simulink model "Record_accelerometer"  (R2014a)
settings: Solver=FixedStepDiscrete  StartTime=0.0  StopTime=300  FixedStep=1/400  RelTol=1e-3
undefined symbols (not defined in the file or in its folder): DiscIntNeverNeededParam
libraries: simulink x6, aerolibtransform2 x4, vrlib x3, aerolibutil x2, AR_Drone_2_Library x1, dspmtrx3 x1, Navigation_Lib x1
(part 1 of 2)
settings Model: SimulationMode=external  ExtModeTrigDuration=120003  Creator=darenlee  LastModifiedBy=darenlee
settings OptimizationCC: OptimizeModelRefInitCode=on  LifeSpan=1  MaxStackSize=64
settings DebuggingCC: UnderspecifiedInitializationDetection=Classic
settings HardwareCC: ProdLargestAtomicInteger=Long  ProdLargestAtomicFloat=Double  ProdEndianess=LittleEndian  ProdHWDeviceType=ARM Compatible->ARM Cortex
settings RTWCC: SystemTargetFile=ert.tlc  TLCOptions=-aInlineSetEventsForThisBaseRateFcn=TLC_FALSE -aSuppressMultiTaskScheduler=TLC_FALSE  TemplateMakefile=ert_default_tmf  Description=Embedded Coder  ProcessScript=ert_make_rtw_hook  Toolchain=Code Sourcery
settings CodeAppCC: IgnoreCustomStorageClasses=off
settings ERTTargetCC: ParMdlRefBuildCompliant=on  CompOptLevelCompliant=on  ConcurrentExecutionCompliant=on  ERTFirstTimeCompliant=on  ModelStepFunctionPrototypeControlCompliant=on  CPPClassGenCompliant=on  ExtMode=on  ExtModeMexArgs='192.168.1.1' 1 17725  InlinedParameterPlacement=Hierarchical

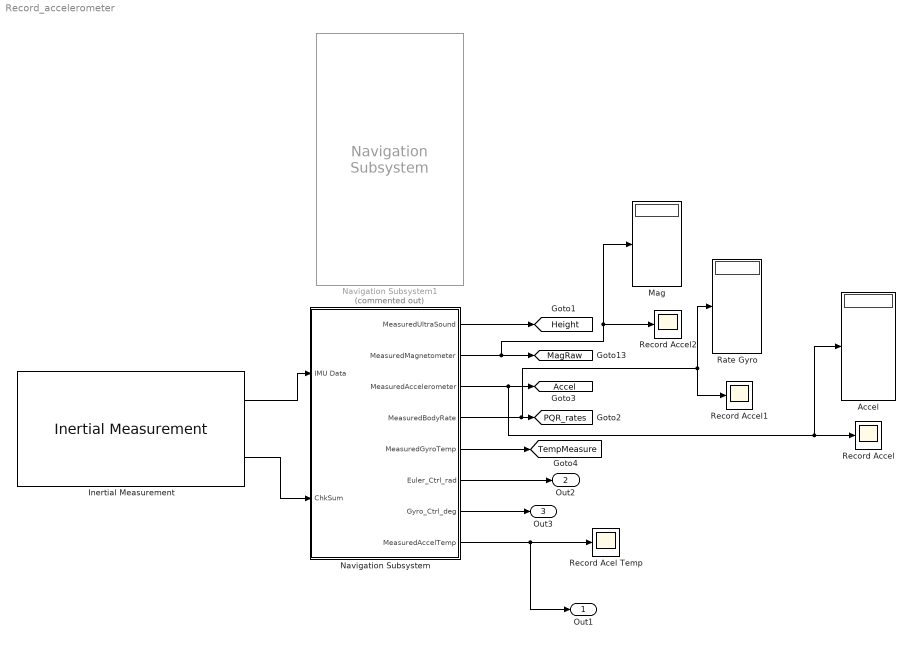
== system Record_accelerometer ==
  Accel : Display
  Inertial Measurement : AR_Drone_2_Library/Inertial Measurement  Ts=1/400
  Mag : Display
  Navigation Subsystem : Subsystem
  Navigation Subsystem1 : Navigation_Lib/Navigation Subsystem  Commented=on  TempProcessVariant=1  PI_YAW_CORRECT=[-0.9 -0.0001]  D_YAW_CORRECT=0  P_GAIN_ROLLPITCH=-2  I_GAIN_ROLLPITCH=-0.01  ACCEL_OFFSET_X=0  ACCEL_OFFSET_Y=0  ACCEL_OFFSET_Z=0
  Rate Gyro : Display
  Record Accel : Scope
      settings: YMin=1550  YMax=2050  SaveName=Accel_Record
  Record Accel1 : Scope
      settings: YMin=1550  YMax=2050  SaveName=Accel_Record1
  Record Accel2 : Scope
      settings: YMin=1550  YMax=2050  SaveName=Accel_Record2
  Record Acel Temp : Scope
      settings: SaveName=Accel_temp
  Out1 : Outport
  Out2 : Outport  Port=2
  Out3 : Outport  Port=3
  tag scope: Accel=global, Height=global, MagRaw=global, PQR_rates=global, TempMeasure=global
  wires:
  Inertial Measurement/1 -> Navigation Subsystem/1(IMU Data)
  Inertial Measurement/2 -> Navigation Subsystem/2(ChkSum)
  Navigation Subsystem/1(MeasuredUltraSound) -> [Height]
  Navigation Subsystem/2(MeasuredMagnetometer) -> Mag/1, Record Accel2/1, [MagRaw]
  Navigation Subsystem/3(MeasuredAccelerometer) -> Accel/1, Record Accel/1, [Accel]
  Navigation Subsystem/4(MeasuredBodyRate) -> Record Accel1/1, Rate Gyro/1, [PQR_rates]
  Navigation Subsystem/5(MeasuredGyroTemp) -> [TempMeasure]
  Navigation Subsystem/8(MeasuredAccelTemp) -> Out1/1, Record Acel Temp/1
  Navigation Subsystem/6(Euler_Ctrl_rad) -> Out2/1
  Navigation Subsystem/7(Gyro_Ctrl_deg) -> Out3/1

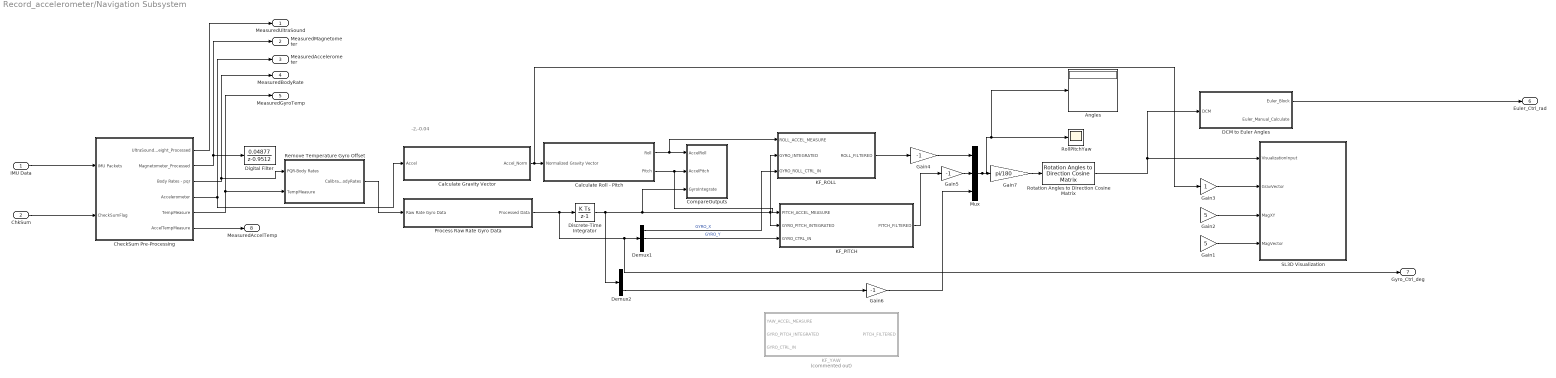
== system Record_accelerometer/Navigation Subsystem ==
  note: -2,-0.04
  IMU Data : Inport
  ChkSum : Inport  Port=2
  Angles : Display
  Calculate Gravity Vector : Subsystem
  Calculate Roll - Pitch : Subsystem
  CheckSum Pre-Processing : Subsystem
  CompareOutputs : Subsystem
  DCM to Euler Angles : Subsystem
  Demux1 : Demux  Outputs=3
  Demux2 : Demux  Outputs=3
  Digital Filter : DiscreteTransferFcn  Numerator=[0.04877]  Denominator=[1 -0.9512]  SampleTime=1/400
  Discrete-Time Integrator : DiscreteIntegrator  SampleTime=1/400  ICPrevOutput=DiscIntNeverNeededParam  ICPrevScaledInput=DiscIntNeverNeededParam
  Gain1 : Gain  Gain=5  OutDataTypeStr=double
  Gain2 : Gain  Gain=5  OutDataTypeStr=double
  Gain3 : Gain  OutDataTypeStr=double
  Gain4 : Gain  Gain=-1
  Gain5 : Gain  Gain=-1
  Gain6 : Gain  Gain=-1
  Gain7 : Gain  Gain=pi/180
  KF_PITCH : Subsystem
  KF_ROLL : Subsystem
  KF_YAW : Subsystem  Commented=on
  Mux : Mux  Inputs=3
  Process Raw Rate Gyro Data : Subsystem
  Remove Temperature Gyro Offset : Subsystem  Variant=on  OverrideUsingVariant=TempConditionA
  RollPitchYaw : Scope
      settings: YMin=0  YMax=70  SaveName=ScopeData15
  Rotation Angles to Direction Cosine Matrix : aerolibtransform2/Rotation Angles to Direction Cosine Matrix  rotationOrder=XYZ
  SL3D Visualization : Subsystem
  MeasuredUltraSound : Outport
  MeasuredMagnetometer : Outport  Port=2
  MeasuredAccelerometer : Outport  Port=3
  MeasuredBodyRate : Outport  Port=4
  MeasuredGyroTemp : Outport  Port=5
  Euler_Ctrl_rad : Outport  Port=6
  Gyro_Ctrl_deg : Outport  Port=7
  MeasuredAccelTemp : Outport  Port=8
  wires:
  IMU Data/1 -> CheckSum Pre-Processing/1(IMU Packets)
  ChkSum/1 -> CheckSum Pre-Processing/2(CheckSumFlag)
  CheckSum Pre-Processing/1(UltraSoundHeight_Processed) -> MeasuredUltraSound/1
  CheckSum Pre-Processing/4(Accelerometer) -> Calculate Gravity Vector/1(Accel), MeasuredAccelerometer/1
  CheckSum Pre-Processing/3(Body Rates - pqr) -> MeasuredBodyRate/1, Remove Temperature Gyro Offset/1(PQR-Body Rates)
  CheckSum Pre-Processing/2(Magnetometer_Processed) -> MeasuredMagnetometer/1, Digital Filter/1
  CheckSum Pre-Processing/5(TempMeasure) -> MeasuredGyroTemp/1, Remove Temperature Gyro Offset/2(TempMeasure)
  Remove Temperature Gyro Offset/1(Calibrated-BodyRates) -> Process Raw Rate Gyro Data/1(Raw Rate Gyro Data)
  Rotation Angles to Direction Cosine Matrix/1 -> SL3D Visualization/1(VisualizationInput), DCM to Euler Angles/1(DCM)
  Gain1/1 -> SL3D Visualization/4(MagVector)
  Gain2/1 -> SL3D Visualization/3(MagXY)
  Calculate Gravity Vector/1(Accel_Norm) -> Gain3/1, Calculate Roll - Pitch/1(Normalized Gravity Vector)
  Gain3/1 -> SL3D Visualization/2(GravVector)
  ? -> Gain1/1
  ? -> Gain2/1
  Mux/1 -> RollPitchYaw/1, Angles/1, Gain7/1
  Process Raw Rate Gyro Data/1(Processed Data) -> Gyro_Ctrl_deg/1, Demux1/1, Discrete-Time Integrator/1
  Calculate Roll - Pitch/1(Roll) -> KF_ROLL/1(ROLL_ACCEL_MEASURE), CompareOutputs/1(AccelRoll)
  Calculate Roll - Pitch/2(Pitch) -> KF_PITCH/1(PITCH_ACCEL_MEASURE), CompareOutputs/2(AccelPitch)
  Discrete-Time Integrator/1 -> CompareOutputs/3(GyroIntegrate), KF_PITCH/2(GYRO_PITCH_INTEGRATED), KF_ROLL/2(GYRO_INTEGRATED), Demux2/1
  Demux1/1 -> KF_ROLL/3(GYRO_ROLL_CTRL_IN)  "GYRO_X"
  Demux1/2 -> KF_PITCH/3(GYRO_CTRL_IN)  "GYRO_Y"
  KF_ROLL/1(ROLL_FILTERED) -> Gain4/1
  KF_PITCH/1(PITCH_FILTERED) -> Gain5/1
  Gain6/1 -> Mux/3
  Gain7/1 -> Rotation Angles to Direction Cosine Matrix/1
  Gain4/1 -> Mux/1
  Gain5/1 -> Mux/2
  Demux2/3 -> Gain6/1
  DCM to Euler Angles/1(Euler_Block) -> Euler_Ctrl_rad/1
  CheckSum Pre-Processing/6(AccelTempMeasure) -> MeasuredAccelTemp/1

== system Record_accelerometer/Navigation Subsystem/Calculate Gravity Vector ==
  Accel : Inport
  Accelerometer Neutral Gain and Offset : Subsystem
  Low Pass Filter : Subsystem
  New Dead Zone Method : Subsystem
  Normalize Vector : vrlib/Utilities/Normalize Vector  Commented=through  maxzero=0
  Old Offset Method : Subsystem
  Scope : Scope
      settings: YMin=-1  YMax=0.05  SaveName=ScopeData11
  Scope1 : Scope  NumInputPorts=2
      settings: TimeRange=6.848856838354834  YMin=-1.05~-1  YMax=0.05~0.05  SaveName=AccelProcessed_Record
  Accel_Norm : Outport
  wires:
  Normalize Vector/1 -> Accel_Norm/1
  Accel/1 -> Accelerometer Neutral Gain and Offset/1(Raw Accel Data)
  Accelerometer Neutral Gain and Offset/1(Processed Accel Data) -> Old Offset Method/1(In1), Scope1/2
  Old Offset Method/1(Out1) -> Scope1/1, Low Pass Filter/1(Offset Accel)
  Low Pass Filter/1(Filtered Accel) -> Normalize Vector/1, Scope/1

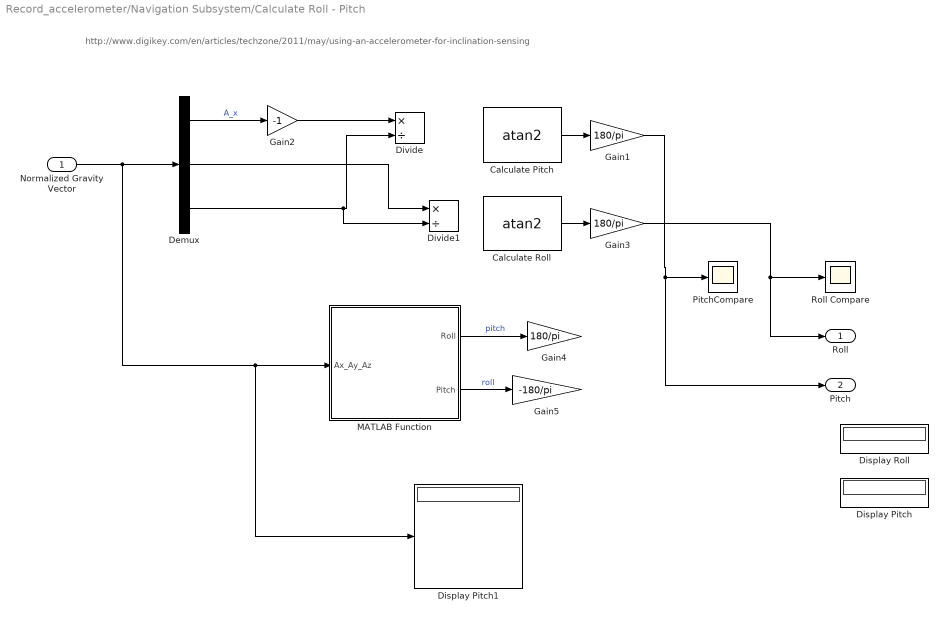
== system Record_accelerometer/Navigation Subsystem/Calculate Roll - Pitch ==
  note: http://www.digikey.com/en/articles/techzone/2011/may/using-an-accelerometer-for-inclination-sensing
  Normalized Gravity Vector : Inport
  Calculate Pitch : Trigonometry  Operator=atan2
  Calculate Roll : Trigonometry  Operator=atan2
  Demux : Demux  Outputs=3
  Display Pitch : Display
  Display Pitch1 : Display
  Display Roll : Display
  Divide : Product  Inputs=*/
  Divide1 : Product  Inputs=*/
  Gain1 : Gain  Gain=180/pi
  Gain2 : Gain  Gain=-1
  Gain3 : Gain  Gain=180/pi
  Gain4 : Gain  Gain=180/pi
  Gain5 : Gain  Gain=-180/pi
  MATLAB Function : MATLAB Function  TreatAsAtomicUnit=on
  PitchCompare : Scope
      settings: YMin=0  YMax=3.25  SaveName=ScopeData9
  Roll Compare : Scope
      settings: TimeRange=30  YMin=-2.175  YMax=-1.7  SaveName=ScopeData5
  Roll : Outport
  Pitch : Outport  Port=2
  wires:
  Calculate Pitch/1 -> Gain1/1
  Calculate Roll/1 -> Gain3/1
  Demux/1 -> Gain2/1  "A_x"
  Normalized Gravity Vector/1 -> Display Pitch1/1, MATLAB Function/1(Ax_Ay_Az), Demux/1
  MATLAB Function/1(Roll) -> Gain4/1  "pitch"
  MATLAB Function/2(Pitch) -> Gain5/1  "roll"
  Gain1/1 -> PitchCompare/1, Pitch/1
  Gain3/1 -> Roll Compare/1, Roll/1
  Demux/2 -> Divide1/1
  Gain2/1 -> Divide/1
  Demux/3 -> Divide1/2, Divide/2

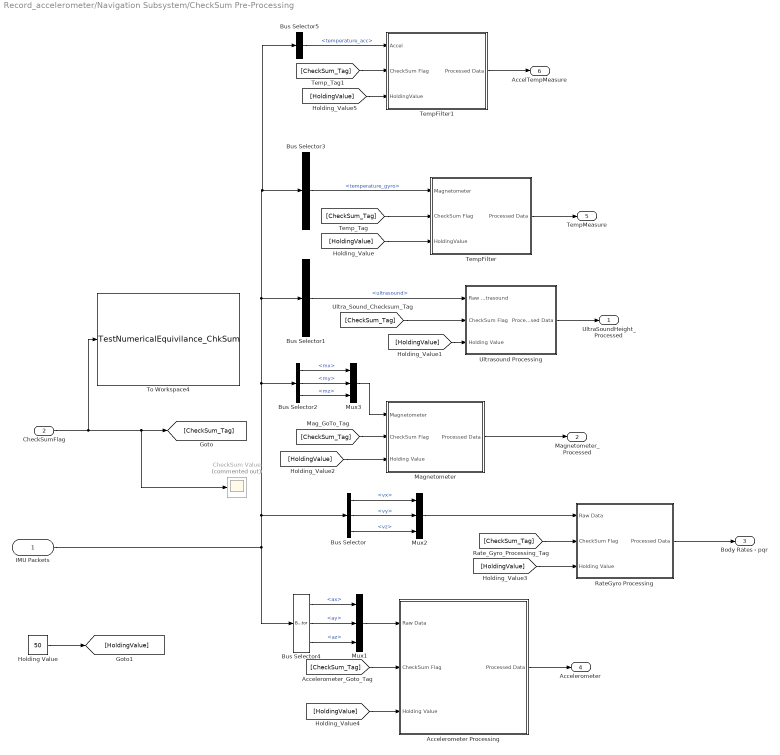
== system Record_accelerometer/Navigation Subsystem/CheckSum Pre-Processing ==
  IMU Packets : Inport
  CheckSumFlag : Inport  Port=2
  Accelerometer Processing : Subsystem
  Bus Selector : BusSelector  OutputSignals=vx,vy,vz
  Bus Selector1 : BusSelector  OutputSignals=ultrasound
  Bus Selector2 : BusSelector  OutputSignals=mx,my,mz
  Bus Selector3 : BusSelector  OutputSignals=temperature_gyro
  Bus Selector4 : BusSelector  OutputSignals=ax,ay,az
  Bus Selector5 : BusSelector  OutputSignals=temperature_acc
  CheckSum Value : Scope  Commented=on
      settings: YMin=0  YMax=2500  SaveName=CheckSum
  Holding Value : Constant  Value=50
  Magnetometer : Subsystem
  Mux1 : Mux  Inputs=3
  Mux2 : Mux  Inputs=3
  Mux3 : Mux  Inputs=3
  RateGyro Processing : Subsystem
  TempFilter : Subsystem
  TempFilter1 : Subsystem
  To Workspace4 : ToWorkspace  VariableName=TestNumericalEquivilance_ChkSum  SaveFormat=Structure With Time  SampleTime=-1
  Ultrasound Processing : Subsystem
  UltraSoundHeight_Processed : Outport
  Magnetometer_Processed : Outport  Port=2
  Body Rates - pqr : Outport  Port=3
  Accelerometer : Outport  Port=4
  TempMeasure : Outport  Port=5
  AccelTempMeasure : Outport  Port=6
  wires:
  Bus Selector1/1 -> Ultrasound Processing/1(Raw Ultrasound)  "<ultrasound>"
  CheckSumFlag/1 -> To Workspace4/1, [CheckSum_Tag], CheckSum Value/1
  IMU Packets/1 -> Bus Selector/1, Bus Selector5/1, Bus Selector3/1, Bus Selector1/1, Bus Selector2/1, Bus Selector4/1
  Bus Selector4/1 -> Mux1/1  "<ax>"
  Bus Selector4/2 -> Mux1/2  "<ay>"
  Bus Selector4/3 -> Mux1/3  "<az>"
  Mux1/1 -> Accelerometer Processing/1(Raw Data)
  [CheckSum_Tag] -> Ultrasound Processing/2(CheckSum Flag)
  Accelerometer Processing/1(Processed Data) -> Accelerometer/1
  Mux2/1 -> RateGyro Processing/1(Raw Data)
  [CheckSum_Tag] -> RateGyro Processing/2(CheckSum Flag)
  RateGyro Processing/1(Processed Data) -> Body Rates - pqr/1
  Bus Selector2/1 -> Mux3/1  "<mx>"
  Bus Selector2/2 -> Mux3/2  "<my>"
  Bus Selector2/3 -> Mux3/3  "<mz>"
  [CheckSum_Tag] -> Magnetometer/2(CheckSum Flag)
  Magnetometer/1(Processed Data) -> Magnetometer_Processed/1
  [CheckSum_Tag] -> Accelerometer Processing/2(CheckSum Flag)
  Ultrasound Processing/1(Processed Data) -> UltraSoundHeight_Processed/1
  Bus Selector/1 -> Mux2/1  "<vx>"
  Bus Selector/2 -> Mux2/2  "<vy>"
  Bus Selector/3 -> Mux2/3  "<vz>"
  Bus Selector3/1 -> TempFilter/1(Magnetometer)  "<temperature_gyro>"
  TempFilter/1(Processed Data) -> TempMeasure/1
  [CheckSum_Tag] -> TempFilter/2(CheckSum Flag)
  [HoldingValue] -> TempFilter/3(HoldingValue)
  [HoldingValue] -> Ultrasound Processing/3(Holding Value)
  [HoldingValue] -> Magnetometer/3(Holding Value)
  [HoldingValue] -> RateGyro Processing/3(Holding Value)
  [HoldingValue] -> Accelerometer Processing/3(Holding Value)
  Holding Value/1 -> [HoldingValue]
  Mux3/1 -> Magnetometer/1(Magnetometer)
  TempFilter1/1(Processed Data) -> AccelTempMeasure/1
  [CheckSum_Tag] -> TempFilter1/2(CheckSum Flag)
  [HoldingValue] -> TempFilter1/3(HoldingValue)
  Bus Selector5/1 -> TempFilter1/1(Accel)  "<temperature_acc>"

== system Record_accelerometer/Navigation Subsystem/CompareOutputs ==
  AccelRoll : Inport
  AccelPitch : Inport  Port=2
  GyroIntegrate : Inport  Port=3
  Demux : Demux  Outputs=3
  Mux : Mux  Inputs=2
  Mux1 : Mux  Inputs=2
  Scope : Scope
      settings: YMin=-3  YMax=14  SaveName=ScopeData7
  Scope1 : Scope
      settings: SaveName=ScopeData8
  wires:
  AccelPitch/1 -> Mux1/1
  Demux/2 -> Mux1/2
  AccelRoll/1 -> Mux/1
  Demux/1 -> Mux/2
  GyroIntegrate/1 -> Demux/1
  Mux/1 -> Scope/1
  Mux1/1 -> Scope1/1

== system Record_accelerometer/Navigation Subsystem/DCM to Euler Angles ==
  note: Euler Rotation Order:
      | With the camera facing towards you
      | ______________
      |       Camera          |
      | 1                    2    |
      |                             |
      | 3                    4    |
      | ______________|
      |
      | Rotation
      |
      | Roll+ , increase 2+4
      | Roll - , increase 1 3
      |
      | Pitch+ , increaes 1+2
      | Pitch- , increase 3+4
  DCM : Inport
  Constant2 : Constant  Value=[1 0 0]
  Direction Cosine Matrix to Rotation Angles : aerolibtransform2/Direction Cosine Matrix to Rotation Angles  rotationOrder=XYZ  lim=Default
      settings: AttributesFormatString=Rotation Order: %<rotationOrder>
  EulerAnglesCalculation : Subsystem  TreatAsAtomicUnit=on
  Product : Product  Multiplication=Matrix(*)
  VectorTrace : Scope
      settings: SaveName=RotationVectorTrace
  Euler_Block : Outport
  Euler_Manual_Calculate : Outport  Port=2
  wires:
  DCM/1 -> Direction Cosine Matrix to Rotation Angles/1, Product/1, EulerAnglesCalculation/1(DCM)
  EulerAnglesCalculation/1(Euler Angles) -> Euler_Manual_Calculate/1
  Direction Cosine Matrix to Rotation Angles/1 -> Euler_Block/1
  Constant2/1 -> Product/2
  Product/1 -> VectorTrace/1

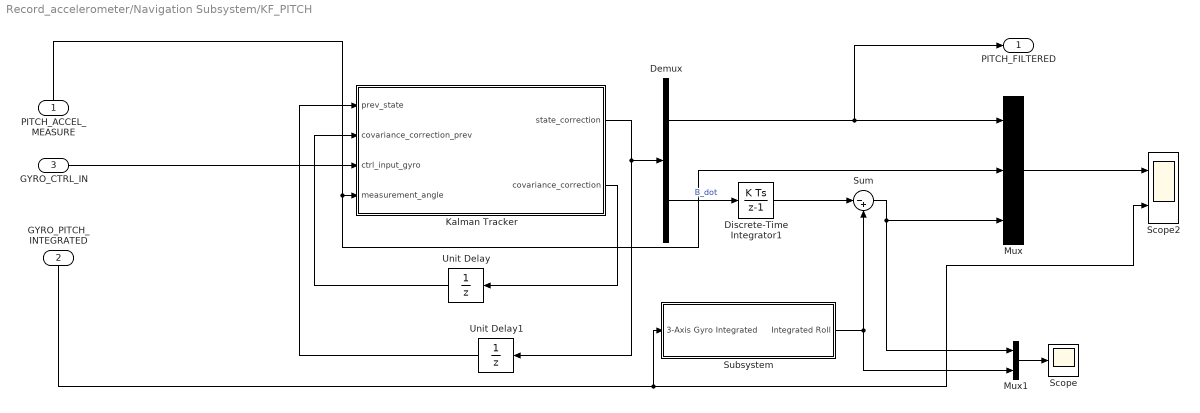
== system Record_accelerometer/Navigation Subsystem/KF_PITCH ==
  PITCH_ACCEL_MEASURE : Inport
  GYRO_PITCH_INTEGRATED : Inport  Port=2
  GYRO_CTRL_IN : Inport  Port=3
  Demux : Demux  Outputs=2
  Discrete-Time Integrator1 : DiscreteIntegrator  SampleTime=1/400  ICPrevOutput=DiscIntNeverNeededParam  ICPrevScaledInput=DiscIntNeverNeededParam
  Kalman Tracker : MATLAB Function  TreatAsAtomicUnit=on
  Mux : Mux  Inputs=3
  Mux1 : Mux  Inputs=2
  Scope : Scope
      settings: YMin=0.05  YMax=1.05  SaveName=ScopeData14
  Scope2 : Scope  NumInputPorts=2
      settings: YMin=0~-90  YMax=30~5  SaveName=ScopeData10
  Subsystem : Subsystem
  Sum : Sum  Inputs=|-+
  Unit Delay : UnitDelay  InitialCondition=eye(2)  SampleTime=-1
  Unit Delay1 : UnitDelay  InitialCondition=[0 0]'  SampleTime=-1
  PITCH_FILTERED : Outport
  wires:
  Mux1/1 -> Scope/1
  Discrete-Time Integrator1/1 -> Sum/1
  Demux/2 -> Discrete-Time Integrator1/1  "B_dot"
  Sum/1 -> Mux1/1, Mux/3
  Subsystem/1(Integrated Roll) -> Mux1/2, Sum/2
  Kalman Tracker/2(covariance_correction) -> Unit Delay/1
  Demux/1 -> PITCH_FILTERED/1, Mux/1
  Kalman Tracker/1(state_correction) -> Unit Delay1/1, Demux/1
  Mux/1 -> Scope2/1
  Unit Delay1/1 -> Kalman Tracker/1(prev_state)
  GYRO_CTRL_IN/1 -> Kalman Tracker/3(ctrl_input_gyro)
  Unit Delay/1 -> Kalman Tracker/2(covariance_correction_prev)
  GYRO_PITCH_INTEGRATED/1 -> Scope2/2, Subsystem/1(3-Axis Gyro Integrated)
  PITCH_ACCEL_MEASURE/1 -> Mux/2, Kalman Tracker/4(measurement_angle)

== system Record_accelerometer/Navigation Subsystem/KF_ROLL ==
  ROLL_ACCEL_MEASURE : Inport
  GYRO_INTEGRATED : Inport  Port=2
  GYRO_ROLL_CTRL_IN : Inport  Port=3
  Demux : Demux  Outputs=2
  Discrete-Time Integrator1 : DiscreteIntegrator  SampleTime=1/400  ICPrevOutput=DiscIntNeverNeededParam  ICPrevScaledInput=DiscIntNeverNeededParam
  Kalman Tracker : MATLAB Function  TreatAsAtomicUnit=on
  Mux : Mux  Inputs=3
  Mux1 : Mux  Inputs=2
  Scope : Scope
      settings: YMin=0.05  YMax=1.05  SaveName=ScopeData14
  Scope2 : Scope  NumInputPorts=2
      settings: YMin=-20.1~-15  YMax=-18~1  SaveName=ScopeData10
  Subsystem : Subsystem
  Sum : Sum  Inputs=|-+
  Unit Delay : UnitDelay  InitialCondition=eye(2)  SampleTime=-1
  Unit Delay1 : UnitDelay  InitialCondition=[0 0]'  SampleTime=-1
  ROLL_FILTERED : Outport
  wires:
  Mux1/1 -> Scope/1
  Discrete-Time Integrator1/1 -> Sum/1
  Demux/2 -> Discrete-Time Integrator1/1  "B_dot"
  Sum/1 -> Mux1/1, Mux/3
  Subsystem/1(Integrated Roll) -> Mux1/2, Sum/2
  Kalman Tracker/2(covariance_correction) -> Unit Delay/1
  Kalman Tracker/1(state_correction) -> Unit Delay1/1, Demux/1
  Mux/1 -> Scope2/1
  Unit Delay1/1 -> Kalman Tracker/1(prev_state)
  GYRO_ROLL_CTRL_IN/1 -> Kalman Tracker/3(ctrl_input_gyro)
  Unit Delay/1 -> Kalman Tracker/2(covariance_correction_prev)
  GYRO_INTEGRATED/1 -> Scope2/2, Subsystem/1(3-Axis Gyro Integrated)
  ROLL_ACCEL_MEASURE/1 -> Mux/2, Kalman Tracker/4(measurement_angle)
  Demux/1 -> ROLL_FILTERED/1, Mux/1

== system Record_accelerometer/Navigation Subsystem/KF_YAW ==
  YAW_ACCEL_MEASURE : Inport
  GYRO_PITCH_INTEGRATED : Inport  Port=2
  GYRO_CTRL_IN : Inport  Port=3
  Demux : Demux  Outputs=2
  Discrete-Time Integrator1 : DiscreteIntegrator  SampleTime=1/400  ICPrevOutput=DiscIntNeverNeededParam  ICPrevScaledInput=DiscIntNeverNeededParam
  Kalman Tracker : MATLAB Function  TreatAsAtomicUnit=on
  Mux : Mux  Inputs=3
  Mux1 : Mux  Inputs=2
  Scope : Scope
      settings: YMin=0.05  YMax=1.05  SaveName=ScopeData14
  Scope2 : Scope  NumInputPorts=2
      settings: YMin=0~-90  YMax=30~5  SaveName=ScopeData10
  Subsystem : Subsystem
  Sum : Sum  Inputs=|-+
  Unit Delay : UnitDelay  InitialCondition=eye(2)  SampleTime=-1
  Unit Delay1 : UnitDelay  InitialCondition=[0 0]'  SampleTime=-1
  PITCH_FILTERED : Outport
  wires:
  Mux1/1 -> Scope/1
  Discrete-Time Integrator1/1 -> Sum/1
  Demux/2 -> Discrete-Time Integrator1/1  "B_dot"
  Sum/1 -> PITCH_FILTERED/1, Mux1/1, Mux/3
  Subsystem/1(Integrated Roll) -> Mux1/2, Sum/2
  Kalman Tracker/2(covariance_correction) -> Unit Delay/1
  Demux/1 -> Mux/1
  Kalman Tracker/1(state_correction) -> Unit Delay1/1, Demux/1
  Mux/1 -> Scope2/1
  Unit Delay1/1 -> Kalman Tracker/1(prev_state)
  GYRO_CTRL_IN/1 -> Kalman Tracker/3(ctrl_input_gyro)
  Unit Delay/1 -> Kalman Tracker/2(covariance_correction_prev)
  GYRO_PITCH_INTEGRATED/1 -> Scope2/2, Subsystem/1(3-Axis Gyro Integrated)
  YAW_ACCEL_MEASURE/1 -> Mux/2, Kalman Tracker/4(measurement_angle)

== system Record_accelerometer/Navigation Subsystem/Process Raw Rate Gyro Data ==
  note: const float Sensitivity[ 3 ] = { 0.0609 , 0.0609 , 0.0609 } ;
      | const float Neutral[ 3 ] = { 0.0 , 0.0 , 0.0 } ;
      | const int16_t Offset[ 3 ] = { - 73 , 14 , - 13 } ;
      | const int16_t Noises[ 3 ] = { 35 , 35 , 15 } ;
      |
      | int16_t vRaws[ 3 ] = {
      | Navdata :: IMU :: Gyroscope :: getRawX (),
      | Navdata :: IMU :: Gyroscope :: getRawY (),
      | Navdata :: IMU :: Gyroscope :: getRawZ ()
      | } ;
      |
      | gyroscope[i] = vRaws[i] * Gyroscope :: Sensitivity[i] * M_PI / 180.0 ;
  Raw Rate Gyro Data : Inport
  Constant1 : Constant  Value=0
  Gain : Gain  Gain=[0.0609, 0.0609, 0.0609]
  Sum : Sum  Inputs=|++
  Processed Data : Outport
  wires:
  Sum/1 -> Gain/1
  Gain/1 -> Processed Data/1
  Raw Rate Gyro Data/1 -> Sum/1
  Constant1/1 -> Sum/2

== system Record_accelerometer/Navigation Subsystem/Remove Temperature Gyro Offset ==
  note: 1) Only subsystems can be added as variant choices at this level
      | 2) Blocks cannot be connected at this level as connectivity is
      | automatically determined at simulation, based on the active variant
  PQR-Body Rates : Inport
  TempMeasure : Inport  Port=2
  TemperatureOffset (home_330453) : Subsystem  VariantControl=TempConditionA
  TemperatureOffset (work_255725) : Subsystem  VariantControl=TempConditionB
  Calibrated-BodyRates : Outport

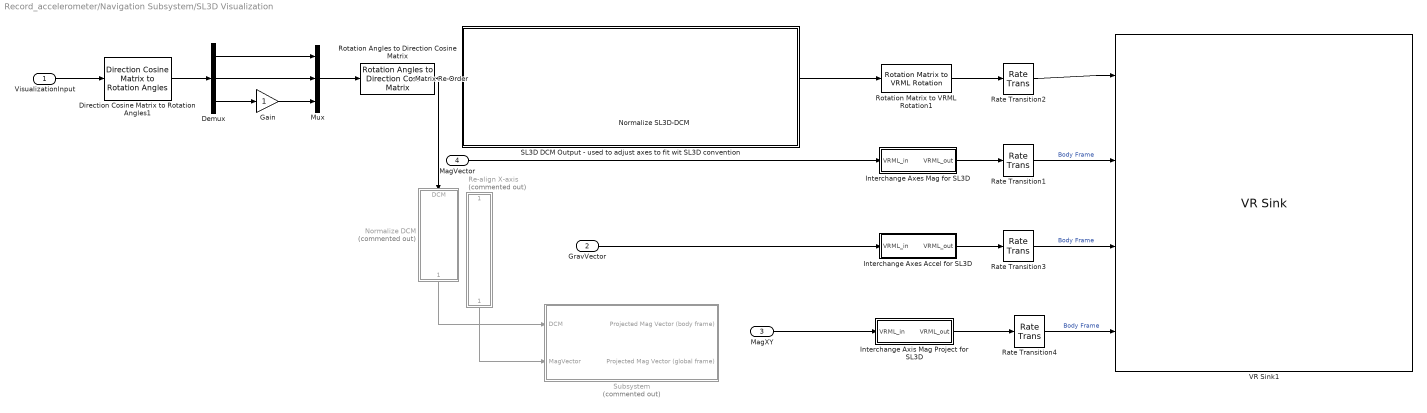
== system Record_accelerometer/Navigation Subsystem/SL3D Visualization ==
  VisualizationInput : Inport
  GravVector : Inport  Port=2
  MagXY : Inport  Port=3
  MagVector : Inport  Port=4
  Demux : Demux  Outputs=3
  Direction Cosine Matrix to Rotation Angles1 : aerolibtransform2/Direction Cosine Matrix to Rotation Angles  rotationOrder=XYZ  lim=ZeroR3
      settings: AttributesFormatString=Rotation Order: %<rotationOrder>
  Gain : Gain  OutDataTypeStr=Inherit: Same as input
  "Interchange Axes Accel for SL3D " : Subsystem
  "Interchange Axes Mag for SL3D " : Subsystem
  Interchange Axis Mag Project for SL3D : Subsystem
  Matrix Re-Order : MATLAB Function  TreatAsAtomicUnit=on
  Mux : Mux  Inputs=3
  Normalize DCM : Subsystem  Commented=on  TreatAsAtomicUnit=on
  Normalize SL3D-DCM : Subsystem  TreatAsAtomicUnit=on
  Rate Transition{1..4} (4 alike) : RateTransition
  Re-align X-axis : Subsystem  Commented=on
  Rotation Angles to Direction Cosine Matrix : aerolibtransform2/Rotation Angles to Direction Cosine Matrix  rotationOrder=XYZ
  Rotation Matrix to VRML Rotation1 : vrlib/Utilities/Rotation Matrix to VRML Rotation  maxzero=1e-12
  SL3D DCM Output - used to adjust axes to fit wit SL3D convention : Subsystem
  Subsystem : Subsystem  Commented=on
  VR Sink1 : vrlib/VR Sink  InstantiateOnLoad=on  SampleTime=0.02  ViewEnable=on  RemoteChange=off  RemoteView=off  FieldsWritten=Plane.rotation.4.1.1.double#mag_point.translation.3.1.1.double#grav_point.translation.3.1.1.double#mag_projection_point.translation.3.1.1.double  WorldFileName=vrml8_grav_2.WRL  AutoView=off  VideoDimensions=[]  AllowVariableSize=off
  wires:
  Rotation Matrix to VRML Rotation1/1 -> Rate Transition2/1
  "Interchange Axes Accel for SL3D "/1(VRML_out) -> Rate Transition3/1
  VisualizationInput/1 -> Direction Cosine Matrix to Rotation Angles1/1
  GravVector/1 -> "Interchange Axes Accel for SL3D "/1(VRML_in)
  Matrix Re-Order/1(M_out) -> Normalize SL3D-DCM/1(DCM)
  Normalize SL3D-DCM/1(DCM_normalized) -> Rotation Matrix to VRML Rotation1/1
  Direction Cosine Matrix to Rotation Angles1/1 -> Demux/1
  Demux/1 -> Mux/1
  Demux/2 -> Mux/2
  Demux/3 -> Gain/1
  Gain/1 -> Mux/3
  Mux/1 -> Rotation Angles to Direction Cosine Matrix/1
  "Interchange Axes Mag for SL3D "/1(VRML_out) -> Rate Transition1/1
  MagVector/1 -> "Interchange Axes Mag for SL3D "/1(VRML_in)
  Rotation Angles to Direction Cosine Matrix/1 -> Matrix Re-Order/1(M_in), Normalize DCM/1(DCM)
  Interchange Axis Mag Project for SL3D/1(VRML_out) -> Rate Transition4/1
  Rate Transition4/1 -> VR Sink1/4  "Body Frame"
  Rate Transition3/1 -> VR Sink1/3  "Body Frame"
  Rate Transition1/1 -> VR Sink1/2  "Body Frame"
  Rate Transition2/1 -> VR Sink1/1
  Normalize DCM/1(DCM_normalized) -> Subsystem/1(DCM)
  Re-align X-axis/1(MagVectorOut) -> Subsystem/2(MagVector)
  MagXY/1 -> Interchange Axis Mag Project for SL3D/1(VRML_in)

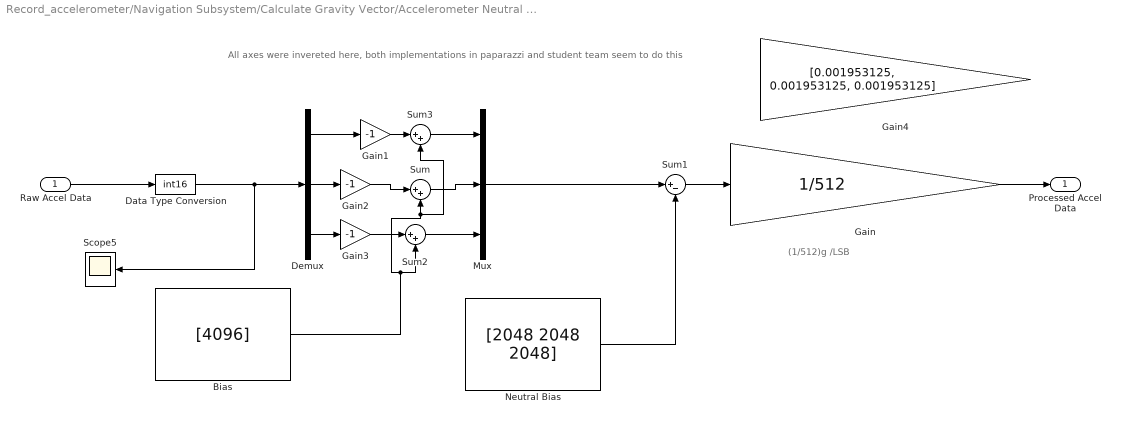
== system Record_accelerometer/Navigation Subsystem/Calculate Gravity Vector/Accelerometer Neutral Gain and Offset ==
  note: All axes were invereted here, both implementations in paparazzi and student team seem to do this
  note: (1/512)g /LSB
  Raw Accel Data : Inport
  Bias : Constant  Value=[4096]
  Data Type Conversion : DataTypeConversion  OutDataTypeStr=int16
  Demux : Demux  Outputs=3
  Gain : Gain  Gain=1/512
  Gain1 : Gain  Gain=-1  OutDataTypeStr=double
  Gain2 : Gain  Gain=-1  OutDataTypeStr=double
  Gain3 : Gain  Gain=-1  OutDataTypeStr=double
  Gain4 : Gain  Gain=[0.001953125, 0.001953125, 0.001953125]
  Mux : Mux  Inputs=3
  Neutral Bias : Constant  Value=[2048 2048 2048]
  Scope5 : Scope
      settings: TimeRange=40  YMin=1530.554926387316  YMax=2010.554926387316  SaveName=ScopeData6
  Sum : Sum  Inputs=|++
  Sum1 : Sum  Inputs=|+-
  Sum2 : Sum  Inputs=|++
  Sum3 : Sum  Inputs=|++
  Processed Accel Data : Outport
  wires:
  Sum1/1 -> Gain/1
  Gain/1 -> Processed Accel Data/1
  Mux/1 -> Sum1/1
  Neutral Bias/1 -> Sum1/2
  Raw Accel Data/1 -> Data Type Conversion/1
  Demux/1 -> Gain1/1
  Sum3/1 -> Mux/1
  Demux/2 -> Gain2/1
  Gain2/1 -> Sum/1
  Sum/1 -> Mux/2
  Demux/3 -> Gain3/1
  Gain3/1 -> Sum2/1
  Sum2/1 -> Mux/3
  Bias/1 -> Sum2/2, Sum3/2, Sum/2
  Data Type Conversion/1 -> Scope5/1, Demux/1
  Gain1/1 -> Sum3/1

== system Record_accelerometer/Navigation Subsystem/Calculate Gravity Vector/Low Pass Filter ==
  Offset Accel : Inport
  Add : Sum
  Gain : Gain  Gain=0.8
  Gain1 : Gain  Gain=0.2
  Unit Delay : UnitDelay  SampleTime=-1
  Filtered Accel : Outport
  wires:
  Unit Delay/1 -> Gain/1
  Gain1/1 -> Add/1
  Gain/1 -> Add/2
  Add/1 -> Unit Delay/1, Filtered Accel/1
  Offset Accel/1 -> Gain1/1

== system Record_accelerometer/Navigation Subsystem/Calculate Gravity Vector/New Dead Zone Method ==
  note: For Work Drone
  In1 : Inport
  Constant3 : Constant  Value=0.0306
  Constant4 : Constant  Value=-0.04
  Constant5 : Constant  Value=- 0.0034
  Dead Zone : DeadZone  LowerValue=-0.04  UpperValue=0.04  SaturateOnIntegerOverflow=on
  Display : Display
  Display1 : Display
  Out1 : Outport
  wires:
  In1/1 -> Dead Zone/1, Display/1
  Constant3/1 -> ?
  Constant5/1 -> ?
  Constant4/1 -> ?
  Dead Zone/1 -> Display1/1, Out1/1

== system Record_accelerometer/Navigation Subsystem/Calculate Gravity Vector/Old Offset Method ==
  note: For Work Drone
  note: For Home Drone
  In1 : Inport
  Constant : Constant  Value=0.015
  Constant1 : Constant  Value=0.0078
  Constant2 : Constant  Value=-0.02
  Constant3 : Constant  Value=0.0306
  Constant4 : Constant  Value=-0.04
  Constant5 : Constant  Value=- 0.0034
  Demux : Demux  Outputs=3
  Display : Display
  Display1 : Display
  Mux1 : Mux  Inputs=3
  Sum : Sum  Inputs=|++
  Sum1 : Sum  Inputs=|++
  Sum2 : Sum  Inputs=|++
  Out1 : Outport
  wires:
  Constant4/1 -> ?
  Constant5/1 -> ?
  Constant3/1 -> ?
  Sum/1 -> Mux1/1
  Sum2/1 -> Mux1/3
  In1/1 -> Demux/1, Display/1
  Demux/3 -> Sum2/1
  Constant1/1 -> Sum1/2
  Sum1/1 -> Mux1/2
  Constant2/1 -> Sum2/2
  Demux/1 -> Sum/1
  Constant/1 -> Sum/2
  Demux/2 -> Sum1/1
  Mux1/1 -> Out1/1, Display1/1

== system Record_accelerometer/Navigation Subsystem/CheckSum Pre-Processing/Accelerometer Processing ==
  Raw Data : Inport
  CheckSum Flag : Inport  Port=2
  Holding Value : Inport  Port=3
  Calculate Accel Data : Subsystem  Commented=through
  CheckSum Correction : Subsystem
  Processed Data : Outport
  wires:
  CheckSum Flag/1 -> CheckSum Correction/2(CheckSumFlag)
  Raw Data/1 -> Calculate Accel Data/1(Raw Accel Data)
  CheckSum Correction/1(Pre-Processed Height) -> Processed Data/1
  Calculate Accel Data/1(Processed Accel Data) -> CheckSum Correction/1(CalculatedData)
  Holding Value/1 -> CheckSum Correction/3(Holding Value)

== system Record_accelerometer/Navigation Subsystem/CheckSum Pre-Processing/Magnetometer ==
  Magnetometer : Inport
  CheckSum Flag : Inport  Port=2
  Holding Value : Inport  Port=3
  CheckSum Correction : Subsystem
  Display : Display
  Process Raw Mag Data : Subsystem  Commented=through
  Processed Data : Outport
  wires:
  CheckSum Flag/1 -> CheckSum Correction/2(CheckSumFlag)
  CheckSum Correction/1(Pre-Processed Data) -> Display/1, Processed Data/1
  Magnetometer/1 -> Process Raw Mag Data/1(Magnetometer)
  Process Raw Mag Data/1(ProcessedData) -> CheckSum Correction/1(CalculatedData)
  Holding Value/1 -> CheckSum Correction/3(Holding Value)

== system Record_accelerometer/Navigation Subsystem/CheckSum Pre-Processing/RateGyro Processing ==
  Raw Data : Inport
  CheckSum Flag : Inport  Port=2
  Holding Value : Inport  Port=3
  CheckSum Correction : Subsystem
  Process Data : Subsystem  Commented=through
  Processed Data : Outport
  wires:
  CheckSum Flag/1 -> CheckSum Correction/2(CheckSumFlag)
  CheckSum Correction/1(Pre-Processed Height) -> Processed Data/1
  Raw Data/1 -> Process Data/1(Raw Data)
  Process Data/1(Processed Data) -> CheckSum Correction/1(CalculatedData)
  Holding Value/1 -> CheckSum Correction/3(Holding Value)

== system Record_accelerometer/Navigation Subsystem/CheckSum Pre-Processing/TempFilter ==
  Magnetometer : Inport
  CheckSum Flag : Inport  Port=2
  HoldingValue : Inport  Port=3
  CheckSum Correction : Subsystem
  Display : Display
  Process Raw Mag Data : Subsystem  Commented=through
  Processed Data : Outport
  wires:
  CheckSum Flag/1 -> CheckSum Correction/2(CheckSumFlag)
  CheckSum Correction/1(Pre-Processed Data) -> Display/1, Processed Data/1
  Magnetometer/1 -> Process Raw Mag Data/1(Magnetometer)
  Process Raw Mag Data/1(ProcessedData) -> CheckSum Correction/1(CalculatedData)
  HoldingValue/1 -> CheckSum Correction/3(Holding Value)

== system Record_accelerometer/Navigation Subsystem/CheckSum Pre-Processing/TempFilter1 ==
  Accel : Inport
  CheckSum Flag : Inport  Port=2
  HoldingValue : Inport  Port=3
  CheckSum Correction : Subsystem
  Display : Display
  Process Raw Mag Data : Subsystem  Commented=through
  Processed Data : Outport
  wires:
  CheckSum Flag/1 -> CheckSum Correction/2(CheckSumFlag)
  CheckSum Correction/1(Pre-Processed Data) -> Display/1, Processed Data/1
  Accel/1 -> Process Raw Mag Data/1(Magnetometer)
  Process Raw Mag Data/1(ProcessedData) -> CheckSum Correction/1(CalculatedData)
  HoldingValue/1 -> CheckSum Correction/3(Holding Value)

== system Record_accelerometer/Navigation Subsystem/CheckSum Pre-Processing/Ultrasound Processing ==
  note: '192.168.1.1' 1 17725
  Raw Ultrasound : Inport
  CheckSum Flag : Inport  Port=2
  Holding Value : Inport  Port=3
  CheckSum Correction : Subsystem
  Data Type Conversion1 : DataTypeConversion
  Delay1 : Delay  DelayLength=1  InitialCondition=0
  Display : Display
  Height Calculation : MATLAB Function  TreatAsAtomicUnit=on
  Saturation1 : Saturate  UpperLimit=100e3  LowerLimit=0
  Processed Data : Outport
  wires:
  Delay1/1 -> Height Calculation/2(z_1)
  Data Type Conversion1/1 -> Height Calculation/1(u)
  Height Calculation/2(prev_good_height) -> Delay1/1
  Raw Ultrasound/1 -> Data Type Conversion1/1
  Height Calculation/1(y) -> CheckSum Correction/1(CalculatedData)
  CheckSum Flag/1 -> CheckSum Correction/2(CheckSumFlag)
  CheckSum Correction/1(Pre-Processed Height) -> Display/1, Saturation1/1
  Saturation1/1 -> Processed Data/1
  Holding Value/1 -> CheckSum Correction/3(Holding Value)

== system Record_accelerometer/Navigation Subsystem/DCM to Euler Angles/EulerAnglesCalculation ==
  DCM : Inport
  Demux : Demux  Outputs=2
  Demux1 : Demux  Outputs=2
  Gain : Gain  Gain=-1
  Gain1 : Gain  OutDataTypeStr=Inherit: Same as input
  Mux : Mux  Inputs=3
  Selector : Selector  NumberOfDimensions=2  IndexMode=Zero-based  InputPortWidth=3  IndexOptions=Index vector (dialog),Index vector (dialog)  Indices=2,0  OutputSizes=1,1
  Selector1 : Selector  NumberOfDimensions=2  IndexMode=Zero-based  InputPortWidth=3  IndexOptions=Index vector (dialog),Index vector (dialog)  Indices=2,[1 2]  OutputSizes=1,1
  Selector2 : Selector  NumberOfDimensions=2  IndexMode=Zero-based  InputPortWidth=3  IndexOptions=Index vector (dialog),Index vector (dialog)  Indices=[1 0],0  OutputSizes=1,1
  Trigonometric Function : Trigonometry  Operator=asin
  Trigonometric Function1 : Trigonometry  Operator=atan2
  Trigonometric Function2 : Trigonometry  Operator=atan2
  Euler Angles : Outport  InitialOutput=[0 0 0]
  wires:
  Demux1/2 -> Trigonometric Function2/2
  Demux1/1 -> Trigonometric Function2/1
  Mux/1 -> Euler Angles/1
  Selector2/1 -> Demux1/1  "DCM_1_0_DCM_0_0"
  Trigonometric Function2/1 -> Gain1/1  "yaw"
  Trigonometric Function1/1 -> Mux/1  "roll"
  Demux/2 -> Trigonometric Function1/2
  Demux/1 -> Trigonometric Function1/1
  Selector1/1 -> Demux/1  "DCM_2_1_DCM_2_2"
  Trigonometric Function/1 -> Mux/2  "pitch"
  Gain/1 -> Trigonometric Function/1
  Selector/1 -> Gain/1  "DCM_2_0"
  DCM/1 -> Selector/1, Selector2/1, Selector1/1
  Gain1/1 -> Mux/3

== system Record_accelerometer/Navigation Subsystem/KF_PITCH/Subsystem ==
  3-Axis Gyro Integrated : Inport
  Demux2 : Demux  Outputs=3
  Integrated Roll : Outport
  wires:
  Demux2/2 -> Integrated Roll/1  "Roll Axis"
  3-Axis Gyro Integrated/1 -> Demux2/1

== system Record_accelerometer/Navigation Subsystem/KF_ROLL/Subsystem ==
  3-Axis Gyro Integrated : Inport
  Demux2 : Demux  Outputs=3
  Integrated Roll : Outport
  wires:
  Demux2/1 -> Integrated Roll/1  "Roll Axis"
  3-Axis Gyro Integrated/1 -> Demux2/1

== system Record_accelerometer/Navigation Subsystem/KF_YAW/Subsystem ==
  3-Axis Gyro Integrated : Inport
  Demux2 : Demux  Outputs=3
  Integrated Roll : Outport
  wires:
  Demux2/2 -> Integrated Roll/1  "Roll Axis"
  3-Axis Gyro Integrated/1 -> Demux2/1

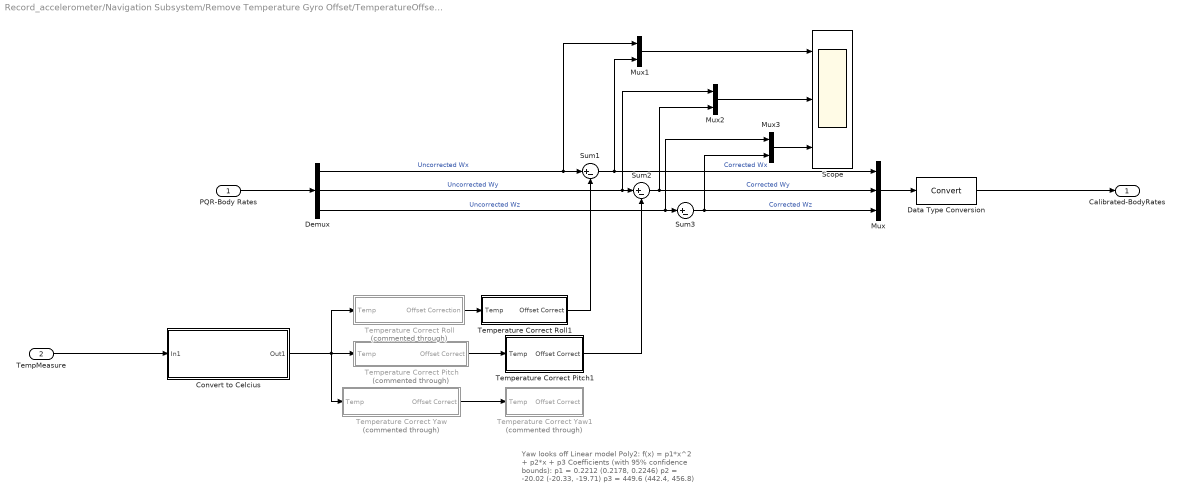
== system Record_accelerometer/Navigation Subsystem/Remove Temperature Gyro Offset/TemperatureOffset (home_330453) ==
  note: Yaw looks off
      |
      | Linear model Poly2:
      |      f(x) = p1*x^2 + p2*x + p3
      | Coefficients (with 95% confidence bounds):
      |        p1 =      0.2212  (0.2178, 0.2246)
      |        p2 =      -20.02  (-20.33, -19.71)
      |        p3 =       449.6  (442.4, 456.8)
  PQR-Body Rates : Inport
  TempMeasure : Inport  Port=2
  Convert to Celcius : Subsystem
  Data Type Conversion : DataTypeConversion
  Demux : Demux  Outputs=3
  Mux : Mux  Inputs=3
  Mux1 : Mux  Inputs=2
  Mux2 : Mux  Inputs=2
  Mux3 : Mux  Inputs=2
  Scope : Scope  NumInputPorts=3
      settings: ShowLegends=on  YMin=-10~-4~-4  YMax=120~11~14  SaveName=TempOffsetCorrect
  Sum1 : Sum  Inputs=|+-
  Sum2 : Sum  Inputs=|+-
  Sum3 : Sum  Inputs=|+-
  Temperature Correct Pitch : Subsystem  Commented=through
  Temperature Correct Pitch1 : Subsystem
  Temperature Correct Roll : Subsystem  Commented=through
  Temperature Correct Roll1 : Subsystem
  Temperature Correct Yaw : Subsystem  Commented=through
  Temperature Correct Yaw1 : Subsystem  Commented=through
  Calibrated-BodyRates : Outport
  wires:
  Sum3/1 -> Mux3/2, Mux/3  "Corrected Wz"
  Demux/2 -> Mux2/1, Sum2/1  "Uncorrected Wy"
  Demux/3 -> Mux3/1, Sum3/1  "Uncorrected Wz"
  Sum1/1 -> Mux1/2, Mux/1  "Corrected Wx"
  Demux/1 -> Mux1/1, Sum1/1  "Uncorrected Wx"
  PQR-Body Rates/1 -> Demux/1
  Mux/1 -> Data Type Conversion/1
  Data Type Conversion/1 -> Calibrated-BodyRates/1
  Sum2/1 -> Mux2/2, Mux/2  "Corrected Wy"
  Mux1/1 -> Scope/1
  Mux2/1 -> Scope/2
  Mux3/1 -> Scope/3
  Temperature Correct Roll/1(Offset Correction) -> Temperature Correct Roll1/1(Temp)
  Temperature Correct Pitch/1(Offset Correct) -> Temperature Correct Pitch1/1(Temp)
  Temperature Correct Yaw/1(Offset Correct) -> Temperature Correct Yaw1/1(Temp)
  TempMeasure/1 -> Convert to Celcius/1(In1)
  Convert to Celcius/1(Out1) -> Temperature Correct Yaw/1(Temp), Temperature Correct Pitch/1(Temp), Temperature Correct Roll/1(Temp)
  Temperature Correct Roll1/1(Offset Correct) -> Sum1/2
  Temperature Correct Pitch1/1(Offset Correct) -> Sum2/2

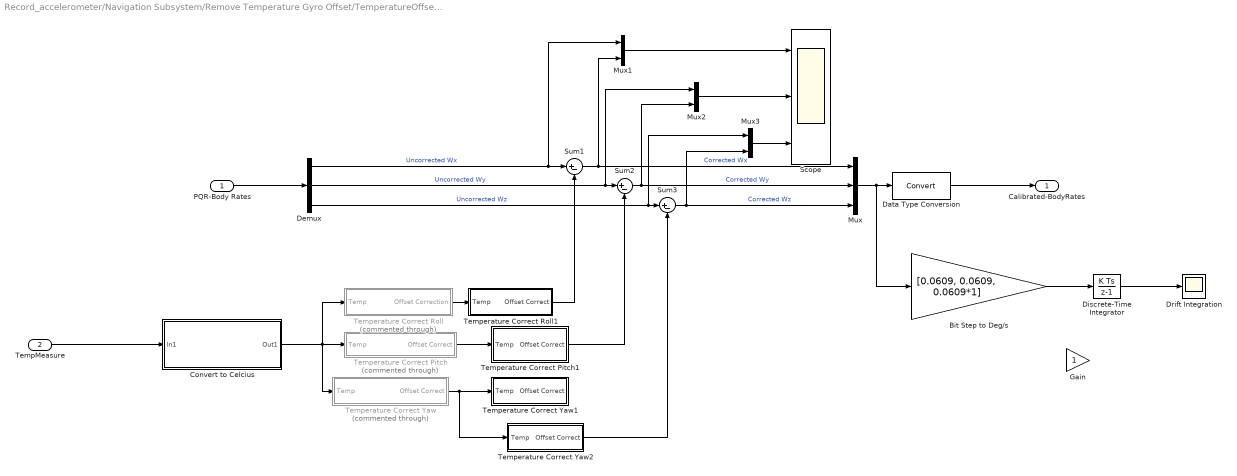
== system Record_accelerometer/Navigation Subsystem/Remove Temperature Gyro Offset/TemperatureOffset (work_255725) ==
  PQR-Body Rates : Inport
  TempMeasure : Inport  Port=2
  Bit Step to Deg/s : Gain  Gain=[0.0609, 0.0609, 0.0609*1]
  Convert to Celcius : Subsystem
  Data Type Conversion : DataTypeConversion
  Demux : Demux  Outputs=3
  Discrete-Time Integrator : DiscreteIntegrator  SampleTime=-1  ICPrevOutput=DiscIntNeverNeededParam  ICPrevScaledInput=DiscIntNeverNeededParam
  Drift Integration : Scope
      settings: YMin=0  YMax=2200  SaveName=ScopeData2
  Gain : Gain
  Mux : Mux  Inputs=3
  Mux1 : Mux  Inputs=2
  Mux2 : Mux  Inputs=2
  Mux3 : Mux  Inputs=2
  Scope : Scope  NumInputPorts=3
      settings: ShowLegends=on  YMin=-5~-12~-15  YMax=90~5~65  SaveName=TempOffsetCorrect
  Sum1 : Sum  Inputs=|+-
  Sum2 : Sum  Inputs=|+-
  Sum3 : Sum  Inputs=|+-
  Temperature Correct Pitch : Subsystem  Commented=through
  Temperature Correct Pitch1 : Subsystem
  Temperature Correct Roll : Subsystem  Commented=through
  Temperature Correct Roll1 : Subsystem
  Temperature Correct Yaw : Subsystem  Commented=through
  Temperature Correct Yaw1 : Subsystem
  Temperature Correct Yaw2 : Subsystem
  Calibrated-BodyRates : Outport
  wires:
  Sum3/1 -> Mux3/2, Mux/3  "Corrected Wz"
  Demux/2 -> Mux2/1, Sum2/1  "Uncorrected Wy"
  Demux/3 -> Mux3/1, Sum3/1  "Uncorrected Wz"
  Sum1/1 -> Mux1/2, Mux/1  "Corrected Wx"
  Demux/1 -> Mux1/1, Sum1/1  "Uncorrected Wx"
  PQR-Body Rates/1 -> Demux/1
  Data Type Conversion/1 -> Calibrated-BodyRates/1
  Sum2/1 -> Mux2/2, Mux/2  "Corrected Wy"
  Mux1/1 -> Scope/1
  Mux2/1 -> Scope/2
  Mux3/1 -> Scope/3
  Temperature Correct Roll/1(Offset Correction) -> Temperature Correct Roll1/1(Temp)
  Temperature Correct Pitch/1(Offset Correct) -> Temperature Correct Pitch1/1(Temp)
  Temperature Correct Yaw/1(Offset Correct) -> Temperature Correct Yaw2/1(Temp), Temperature Correct Yaw1/1(Temp)
  TempMeasure/1 -> Convert to Celcius/1(In1)
  Convert to Celcius/1(Out1) -> Temperature Correct Yaw/1(Temp), Temperature Correct Pitch/1(Temp), Temperature Correct Roll/1(Temp)
  Temperature Correct Roll1/1(Offset Correct) -> Sum1/2
  Temperature Correct Pitch1/1(Offset Correct) -> Sum2/2
  Temperature Correct Yaw2/1(Offset Correct) -> Sum3/2
  Mux/1 -> Bit Step to Deg/s/1, Data Type Conversion/1
  Bit Step to Deg/s/1 -> Discrete-Time Integrator/1
  Discrete-Time Integrator/1 -> Drift Integration/1

== system Record_accelerometer/Navigation Subsystem/SL3D Visualization/Interchange Axes Accel for SL3D  ==
  VRML_in : Inport
  Demux1 : Demux  Outputs=3
  Gain1 : Gain  Gain=3
  Gain2 : Gain
  Gain3 : Gain
  Mux2 : Mux  Inputs=3
  VRML_out : Outport
  wires:
  Gain1/1 -> Demux1/1
  Demux1/1 -> Gain3/1
  Demux1/3 -> Mux2/2
  Gain2/1 -> Mux2/1
  Gain3/1 -> Mux2/3
  Mux2/1 -> VRML_out/1
  Demux1/2 -> Gain2/1
  VRML_in/1 -> Gain1/1

== system Record_accelerometer/Navigation Subsystem/SL3D Visualization/Interchange Axes Mag for SL3D  ==
  VRML_in : Inport
  Home Drone : Subsystem
  Subsystem : Subsystem  Commented=on
  Work Drone : Subsystem
  Work Drone - supposed work drone .. not really : Subsystem
  VRML_out : Outport
  wires:
  VRML_in/1 -> Work Drone/1(In1), Home Drone/1(In1)
  Work Drone/1(Out1) -> VRML_out/1

== system Record_accelerometer/Navigation Subsystem/SL3D Visualization/Interchange Axis Mag Project for SL3D ==
  VRML_in : Inport
  Demux1 : Demux  Outputs=3
  Gain2 : Gain
  Gain3 : Gain
  Mux2 : Mux  Inputs=3
  VRML_out : Outport
  wires:
  VRML_in/1 -> Demux1/1
  Demux1/1 -> Gain3/1
  Demux1/3 -> Mux2/2
  Gain2/1 -> Mux2/1
  Gain3/1 -> Mux2/3
  Mux2/1 -> VRML_out/1
  Demux1/2 -> Gain2/1

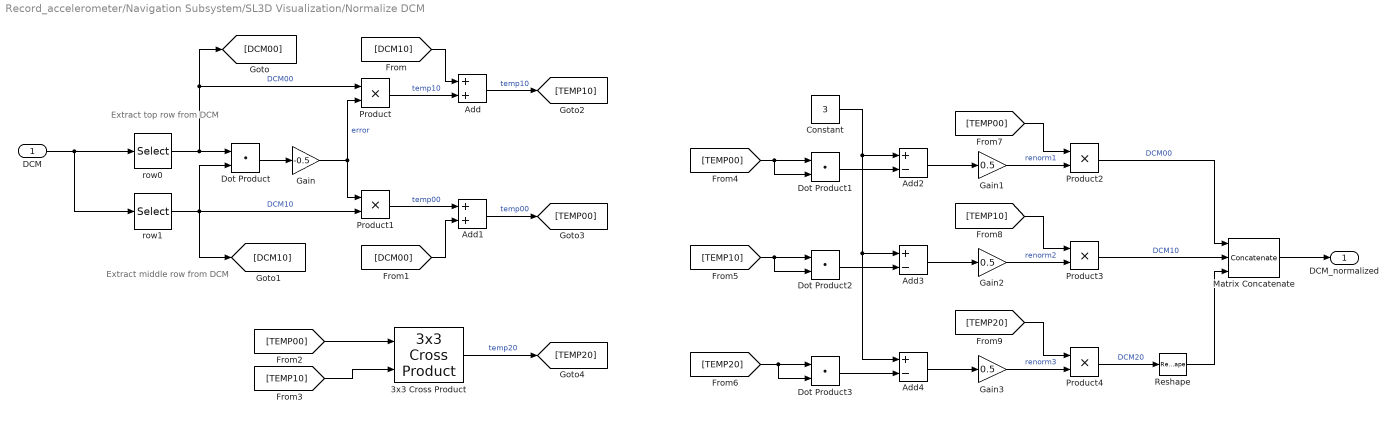
== system Record_accelerometer/Navigation Subsystem/SL3D Visualization/Normalize DCM ==
  note: Extract middle row from DCM
  note: Extract top row from DCM
  DCM : Inport  OutDataTypeStr=double  PortDimensions=[3,3]
  3x3 Cross Product : aerolibutil/3x3 Cross Product
  Add : Sum
  Add1 : Sum
  Add2 : Sum  Inputs=+-
  Add3 : Sum  Inputs=+-
  Add4 : Sum  Inputs=+-
  Constant : Constant  Value=3  OutDataTypeStr=double  SampleTime=-1
  Dot Product{,1..3} (4 alike) : DotProduct  InputSameDT=on  OutDataTypeStr=Inherit: Inherit via internal rule
  Gain : Gain  Gain=-0.5
  Gain1 : Gain  Gain=0.5  OutDataTypeStr=single
  Gain2 : Gain  Gain=0.5  OutDataTypeStr=single
  Gain3 : Gain  Gain=0.5  OutDataTypeStr=single
  Matrix Concatenate : Concatenate  NumInputs=3  Mode=Multidimensional array
  Product{,1..4} (5 alike) : Product  RndMeth=Zero
  Reshape : Reshape  OutputDimensionality=Row vector (2-D)
  row0 : Selector  NumberOfDimensions=2  IndexMode=Zero-based  InputPortWidth=3  IndexOptions=Index vector (dialog),Index vector (dialog)  Indices=0,[0:2]  OutputSizes=1,1
  row1 : Selector  NumberOfDimensions=2  IndexMode=Zero-based  InputPortWidth=3  IndexOptions=Index vector (dialog),Index vector (dialog)  Indices=1,[0:2]  OutputSizes=1,1
  DCM_normalized : Outport  OutDataTypeStr=double
  wires:
  Reshape/1 -> Matrix Concatenate/3
  Matrix Concatenate/1 -> DCM_normalized/1
  Product4/1 -> Reshape/1  "DCM20"
  Product3/1 -> Matrix Concatenate/2  "DCM10"
  Product2/1 -> Matrix Concatenate/1  "DCM00"
  [TEMP20] -> Product4/1
  [TEMP10] -> Product3/1
  [TEMP00] -> Product2/1
  Dot Product3/1 -> Add4/2
  Gain3/1 -> Product4/2  "renorm3"
  Add4/1 -> Gain3/1
  Dot Product2/1 -> Add3/2
  Gain2/1 -> Product3/2  "renorm2"
  Add3/1 -> Gain2/1
  Gain1/1 -> Product2/2  "renorm1"
  Add2/1 -> Gain1/1
  Constant/1 -> Add3/1, Add4/1, Add2/1
  Dot Product1/1 -> Add2/2
  [TEMP20] -> Dot Product3/2, Dot Product3/1
  [TEMP10] -> Dot Product2/2, Dot Product2/1
  [TEMP00] -> Dot Product1/2, Dot Product1/1
  [TEMP10] -> 3x3 Cross Product/2
  [TEMP00] -> 3x3 Cross Product/1
  3x3 Cross Product/1 -> [TEMP20]  "temp20"
  Add1/1 -> [TEMP00]  "temp00"
  Add/1 -> [TEMP10]  "temp10"
  [DCM00] -> Add1/2
  [DCM10] -> Add/1
  Product1/1 -> Add1/1  "temp00"
  Product/1 -> Add/2  "temp10"
  Gain/1 -> Product1/1, Product/2  "error"
  Dot Product/1 -> Gain/1
  row1/1 -> [DCM10], Product1/2, Dot Product/2  "DCM10"
  row0/1 -> [DCM00], Product/1, Dot Product/1  "DCM00"
  DCM/1 -> row1/1, row0/1

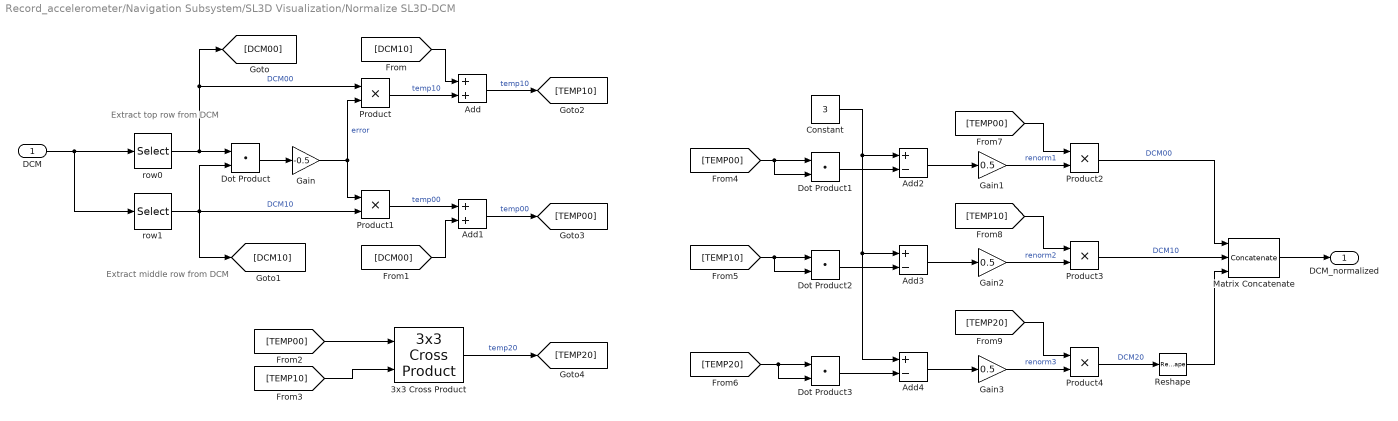
== system Record_accelerometer/Navigation Subsystem/SL3D Visualization/Normalize SL3D-DCM ==
  note: Extract middle row from DCM
  note: Extract top row from DCM
  DCM : Inport  OutDataTypeStr=double  PortDimensions=[3,3]
  3x3 Cross Product : aerolibutil/3x3 Cross Product
  Add : Sum
  Add1 : Sum
  Add2 : Sum  Inputs=+-
  Add3 : Sum  Inputs=+-
  Add4 : Sum  Inputs=+-
  Constant : Constant  Value=3  OutDataTypeStr=double  SampleTime=-1
  Dot Product{,1..3} (4 alike) : DotProduct  InputSameDT=on  OutDataTypeStr=Inherit: Inherit via internal rule
  Gain : Gain  Gain=-0.5
  Gain1 : Gain  Gain=0.5  OutDataTypeStr=single
  Gain2 : Gain  Gain=0.5  OutDataTypeStr=single
  Gain3 : Gain  Gain=0.5  OutDataTypeStr=single
  Matrix Concatenate : Concatenate  NumInputs=3  Mode=Multidimensional array
  Product{,1..4} (5 alike) : Product  RndMeth=Zero
  Reshape : Reshape  OutputDimensionality=Row vector (2-D)
  row0 : Selector  NumberOfDimensions=2  IndexMode=Zero-based  InputPortWidth=3  IndexOptions=Index vector (dialog),Index vector (dialog)  Indices=0,[0:2]  OutputSizes=1,1
  row1 : Selector  NumberOfDimensions=2  IndexMode=Zero-based  InputPortWidth=3  IndexOptions=Index vector (dialog),Index vector (dialog)  Indices=1,[0:2]  OutputSizes=1,1
  DCM_normalized : Outport  OutDataTypeStr=double
  wires:
  Reshape/1 -> Matrix Concatenate/3
  Matrix Concatenate/1 -> DCM_normalized/1
  Product4/1 -> Reshape/1  "DCM20"
  Product3/1 -> Matrix Concatenate/2  "DCM10"
  Product2/1 -> Matrix Concatenate/1  "DCM00"
  [TEMP20] -> Product4/1
  [TEMP10] -> Product3/1
  [TEMP00] -> Product2/1
  Dot Product3/1 -> Add4/2
  Gain3/1 -> Product4/2  "renorm3"
  Add4/1 -> Gain3/1
  Dot Product2/1 -> Add3/2
  Gain2/1 -> Product3/2  "renorm2"
  Add3/1 -> Gain2/1
  Gain1/1 -> Product2/2  "renorm1"
  Add2/1 -> Gain1/1
  Constant/1 -> Add3/1, Add4/1, Add2/1
  Dot Product1/1 -> Add2/2
  [TEMP20] -> Dot Product3/2, Dot Product3/1
  [TEMP10] -> Dot Product2/2, Dot Product2/1
  [TEMP00] -> Dot Product1/2, Dot Product1/1
  [TEMP10] -> 3x3 Cross Product/2
  [TEMP00] -> 3x3 Cross Product/1
  3x3 Cross Product/1 -> [TEMP20]  "temp20"
  Add1/1 -> [TEMP00]  "temp00"
  Add/1 -> [TEMP10]  "temp10"
  [DCM00] -> Add1/2
  [DCM10] -> Add/1
  Product1/1 -> Add1/1  "temp00"
  Product/1 -> Add/2  "temp10"
  Gain/1 -> Product1/1, Product/2  "error"
  Dot Product/1 -> Gain/1
  row1/1 -> [DCM10], Product1/2, Dot Product/2  "DCM10"
  row0/1 -> [DCM00], Product/1, Dot Product/1  "DCM00"
  DCM/1 -> row1/1, row0/1

== system Record_accelerometer/Navigation Subsystem/SL3D Visualization/Re-align X-axis ==
  MagVector : Inport
  Demux1 : Demux  Outputs=3
  Gain : Gain
  Gain1 : Gain  Gain=-1
  Gain2 : Gain
  Mux2 : Mux  Inputs=3
  MagVectorOut : Outport
  wires:
  Mux2/1 -> MagVectorOut/1
  Demux1/1 -> Gain1/1
  Demux1/2 -> Gain2/1
  Demux1/3 -> Gain/1
  Gain1/1 -> Mux2/1
  Gain2/1 -> Mux2/2
  Gain/1 -> Mux2/3
  MagVector/1 -> Demux1/1

== system Record_accelerometer/Navigation Subsystem/SL3D Visualization/SL3D DCM Output - used to adjust axes to fit wit SL3D convention ==

== system Record_accelerometer/Navigation Subsystem/SL3D Visualization/Subsystem ==
  DCM : Inport
  MagVector : Inport  Port=2
  Compensate for Magnetic Declination (~60 degrees in Boston)_ : MATLAB Function  Commented=through  TreatAsAtomicUnit=on
  Compensate for Magnetic Declination (~60 degrees in Boston)_1 : MATLAB Function  TreatAsAtomicUnit=on
  EnlargeVectorAgain : Gain  Commented=through  Gain=3
  Transform MagVector from Body Frame to World Frame : Product  Multiplication=Matrix(*)
  Transform compensated magnetic vector into the  body frame : Product  Multiplication=Matrix(*)
  Transpose2 : dspmtrx3/Transpose  Hermitian=off  overflowFlag=off
  Projected Mag Vector (body frame) : Outport
  Projected Mag Vector (global frame) : Outport  Port=2
  wires:
  MagVector/1 -> EnlargeVectorAgain/1
  Transform compensated magnetic vector into the  body frame/1 -> Projected Mag Vector (body frame)/1
  DCM/1 -> Transpose2/1, Transform MagVector from Body Frame to World Frame/1
  EnlargeVectorAgain/1 -> Transform MagVector from Body Frame to World Frame/2
  Transpose2/1 -> Transform compensated magnetic vector into the  body frame/1
  Transform MagVector from Body Frame to World Frame/1 -> Compensate for Magnetic Declination (~60 degrees in Boston)_/1(vector_in)
  Compensate for Magnetic Declination (~60 degrees in Boston)_/1(y) -> Compensate for Magnetic Declination (~60 degrees in Boston)_1/1(vector_in)
  Compensate for Magnetic Declination (~60 degrees in Boston)_1/1(y) -> Projected Mag Vector (global frame)/1, Transform compensated magnetic vector into the  body frame/2

== system Record_accelerometer/Navigation Subsystem/CheckSum Pre-Processing/Accelerometer Processing/Calculate Accel Data ==
  Raw Accel Data : Inport
  Bias : Constant  Value=[0 4096 4096]
  Gain : Gain  Gain=[0.001953125, 0.001953125, 0.001953125]
  Neutral Bias : Constant  Value=[2048 2048 2048]
  Sum : Sum  Inputs=|-+
  Sum1 : Sum  Inputs=|+-
  Processed Accel Data : Outport
  wires:
  Raw Accel Data/1 -> Sum/1
  Sum1/1 -> Gain/1
  Gain/1 -> Processed Accel Data/1
  Sum/1 -> Sum1/1
  Neutral Bias/1 -> Sum1/2
  Bias/1 -> Sum/2

== system Record_accelerometer/Navigation Subsystem/CheckSum Pre-Processing/Accelerometer Processing/CheckSum Correction ==
  CalculatedData : Inport
  CheckSumFlag : Inport  Port=2
  Holding Value : Inport  Port=3
  Compare To Zero : simulink/Logic and Bit Operations/Compare To Zero  relop=>  OutDataTypeStr=boolean
  Delay : Delay  DelayLength=3  InitialCondition=0
  Generate Sample Holding Pulse : Subsystem
  "If True, we have good data, If false, we have bad data, With bad data, use previous good data from N samples ago and hold it on that value for M samples" : Switch  Criteria=u2 > Threshold
  Invert Logic : Logic  Operator=NOT  AllPortsSameDT=off  OutDataTypeStr=boolean
  Logical Operator1 : Logic  Operator=NOT  AllPortsSameDT=off  OutDataTypeStr=boolean
  Pre-Processed Height : Outport
  wires:
  CheckSumFlag/1 -> Compare To Zero/1
  CalculatedData/1 -> "If True, we have good data, If false, we have bad data, With bad data, use previous good data from N samples ago and hold it on that value for M samples"/1
  "If True, we have good data, If false, we have bad data, With bad data, use previous good data from N samples ago and hold it on that value for M samples"/1 -> Pre-Processed Height/1, Delay/1
  Delay/1 -> "If True, we have good data, If false, we have bad data, With bad data, use previous good data from N samples ago and hold it on that value for M samples"/3
  Compare To Zero/1 -> Logical Operator1/1
  Generate Sample Holding Pulse/1(Hold_Data_Pulse) -> Invert Logic/1
  Logical Operator1/1 -> Generate Sample Holding Pulse/1(CheckSumFlag)
  Invert Logic/1 -> "If True, we have good data, If false, we have bad data, With bad data, use previous good data from N samples ago and hold it on that value for M samples"/2
  Holding Value/1 -> Generate Sample Holding Pulse/2(HoldDataTicks_Value)

== system Record_accelerometer/Navigation Subsystem/CheckSum Pre-Processing/Magnetometer/CheckSum Correction ==
  CalculatedData : Inport
  CheckSumFlag : Inport  Port=2
  Holding Value : Inport  Port=3
  Compare To Zero : simulink/Logic and Bit Operations/Compare To Zero  relop=>  OutDataTypeStr=boolean
  Delay : Delay  DelayLength=3  InitialCondition=0
  Generate Sample Holding Pulse : Subsystem
  "If True, we have good data, If false, we have bad data, With bad data, use previous good data from N samples ago and hold it on that value for M samples" : Switch  Criteria=u2 > Threshold
  Invert Logic : Logic  Operator=NOT  AllPortsSameDT=off  OutDataTypeStr=boolean
  Logical Operator1 : Logic  Operator=NOT  AllPortsSameDT=off  OutDataTypeStr=boolean
  Pre-Processed Data : Outport
  wires:
  CheckSumFlag/1 -> Compare To Zero/1
  CalculatedData/1 -> "If True, we have good data, If false, we have bad data, With bad data, use previous good data from N samples ago and hold it on that value for M samples"/1
  "If True, we have good data, If false, we have bad data, With bad data, use previous good data from N samples ago and hold it on that value for M samples"/1 -> Pre-Processed Data/1, Delay/1
  Delay/1 -> "If True, we have good data, If false, we have bad data, With bad data, use previous good data from N samples ago and hold it on that value for M samples"/3
  Compare To Zero/1 -> Logical Operator1/1
  Generate Sample Holding Pulse/1(Hold_Data_Pulse) -> Invert Logic/1
  Logical Operator1/1 -> Generate Sample Holding Pulse/1(CheckSumFlag)
  Invert Logic/1 -> "If True, we have good data, If false, we have bad data, With bad data, use previous good data from N samples ago and hold it on that value for M samples"/2
  Holding Value/1 -> Generate Sample Holding Pulse/2(HoldDataTicks_Value)

== system Record_accelerometer/Navigation Subsystem/CheckSum Pre-Processing/Magnetometer/Process Raw Mag Data ==
  note: magnetometer[ 0 ] = - ( float ) navdata.mx ;
      | magnetometer[ 1 ] = ( float ) navdata.my ;
      | magnetometer[ 2 ] = - ( float ) navdata.mz ;
      | const float Sensitivity[ 3 ] = { 0.0071492608 , 0.0070882491 , 0.0074057781 } ;
      | const float Neutral[ 3 ] = { 118.0 , - 65.0 , 110.0 } ;
  Magnetometer : Inport
  Bias : Constant  Value=[ 118.0, -65.0, 110.0 ]
  Sum : Sum  Inputs=|+-
  postGain : Gain  Gain=[0.0071492608, 0.0070882491, 0.0074057781]
  preGain : Gain  Gain=[-1 1 -1]
  ProcessedData : Outport
  wires:
  postGain/1 -> ProcessedData/1
  Magnetometer/1 -> preGain/1
  Sum/1 -> postGain/1
  preGain/1 -> Sum/1
  Bias/1 -> Sum/2
